simulink model "sistemaDesacopladoEquivalenteControlTorque"  (R2012b)
settings: Solver=ode45  StartTime=0.0  StopTime=10.0  RelTol=1e-3
values from neighbouring files (symbols this model uses):
  J_m = Jm+(Jl/r^2)    (= 5.65099476805e-06)    [InicializaYconstantes.m]
  lambda = 0.01546    [InicializaYconstantes.m]
  Ld = 6.6*10^-3    (= 0.0066)    [InicializaYconstantes.m]
  Lq = 5.8*10^-3    (= 0.0058)    [InicializaYconstantes.m]
  Pp = 3    [InicializaYconstantes.m]
  R1 = -p1i*Lq    (= 29)    [InicializaYconstantes.m]
  R2 = -p1i*Ld    (= 33)    [InicializaYconstantes.m]
  T_l = Tl/r    (= 0.00499521477515)    [InicializaYconstantes.m]
settings Model: Creator=usuario  LastModifiedBy=usuario

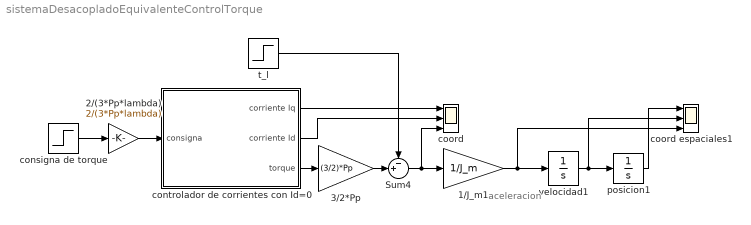
== system sistemaDesacopladoEquivalenteControlTorque ==
  note: aceleracion
  1/J_m1 : Gain  Gain=1/J_m
  2/(3*Pp*lambda) : Gain  Gain=2/(3*Pp*lambda)
  3/2*Pp : Gain  Gain=(3/2)*Pp
  Sum4 : Sum  Inputs=-+|
  consigna de torque : Step  Time=.1  After=.005  SampleTime=0
  controlador de corrientes con Id=0 : Subsystem
  "coord " : Scope  NumInputPorts=3
      settings: TimeRange=10  YMin=0~-1~0  YMax=6~1~0.4  SaveName=ScopeData2  MaxDataPoints=8000
  coord espaciales1 : Scope  NumInputPorts=3
      settings: TimeRange=12  YMin=-1000~0~-50000  YMax=3000~300~100000  SaveName=ScopeData3  MaxDataPoints=8000
  posicion1 : Integrator
  t_l : Step  Time=.3  After=T_l  SampleTime=0
  velocidad1 : Integrator  ContinuousStateAttributes='velocidad'
  wires:
  Sum4/1 -> "coord "/3, 1/J_m1/1
  t_l/1 -> Sum4/1
  1/J_m1/1 -> velocidad1/1, coord espaciales1/3
  posicion1/1 -> coord espaciales1/1
  velocidad1/1 -> posicion1/1, coord espaciales1/2
  consigna de torque/1 -> 2/(3*Pp*lambda)/1
  controlador de corrientes con Id=0/1(corriente Iq) -> "coord "/1
  controlador de corrientes con Id=0/2(corriente Id) -> "coord "/2
  controlador de corrientes con Id=0/3(torque) -> 3/2*Pp/1
  3/2*Pp/1 -> Sum4/2
  2/(3*Pp*lambda)/1 -> controlador de corrientes con Id=0/1(consigna)

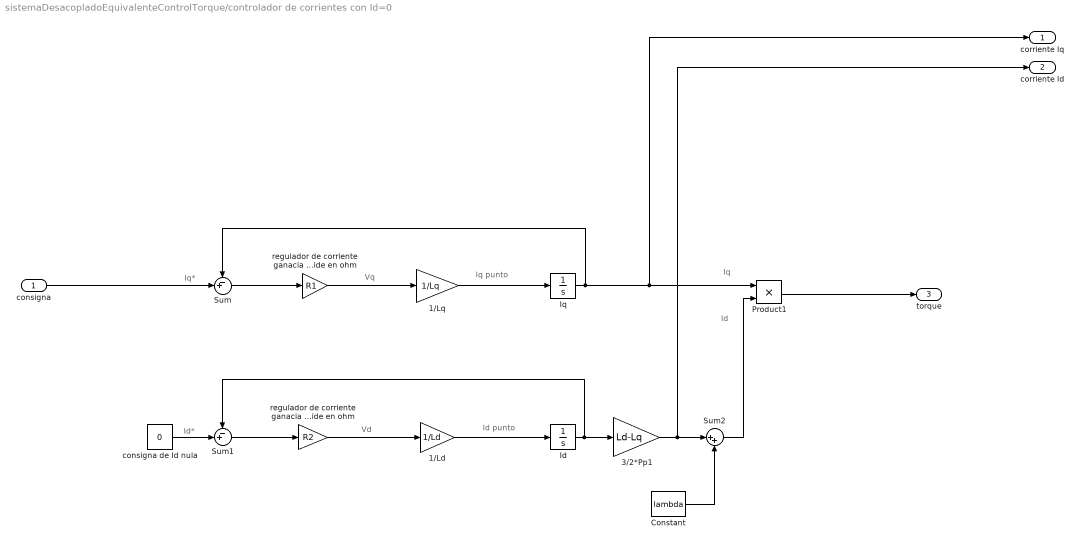
== system sistemaDesacopladoEquivalenteControlTorque/controlador de corrientes con Id=0 ==
  note: Id*
  note: Iq*
  note: Vd
  note: Vq
  note: Iq
  note: Id
  note: Iq punto
  note: Id punto
  consigna : Inport
  1/Ld : Gain  Gain=1/Ld
  1/Lq : Gain  Gain=1/Lq
  3/2*Pp1 : Gain  Gain=Ld-Lq
  Constant : Constant  Value=lambda
  Id : Integrator
  Iq : Integrator
  Product1 : Product  RndMeth=Zero
  Sum : Sum  Inputs=-+|
  Sum1 : Sum  Inputs=-+|
  Sum2 : Sum  Inputs=|++
  consigna de Id nula : Constant  Value=0
  regulador de corriente ganacia proporcional se mide en ohm : Gain  Gain=R2
  regulador de corriente ganacia proporcional1 se mide en ohm : Gain  Gain=R1
  corriente Iq : Outport
  corriente Id : Outport  Port=2
  torque : Outport  Port=3
  wires:
  Product1/1 -> torque/1
  Sum1/1 -> regulador de corriente ganacia proporcional se mide en ohm/1
  consigna de Id nula/1 -> Sum1/2
  Sum/1 -> regulador de corriente ganacia proporcional1 se mide en ohm/1
  Iq/1 -> corriente Iq/1, Product1/1, Sum/1
  1/Ld/1 -> Id/1
  regulador de corriente ganacia proporcional se mide en ohm/1 -> 1/Ld/1
  Id/1 -> Sum1/1, 3/2*Pp1/1
  3/2*Pp1/1 -> corriente Id/1, Sum2/1
  Sum2/1 -> Product1/2
  Constant/1 -> Sum2/2
  regulador de corriente ganacia proporcional1 se mide en ohm/1 -> 1/Lq/1
  1/Lq/1 -> Iq/1
  consigna/1 -> Sum/2
